simulink library "takeoffToLandingOpenWater_cl"  (R2020a)
settings: Solver=VariableStepAuto  StartTime=0.0  StopTime=10.0  RelTol=1e-3
undefined symbols (not defined in the file or in its folder): a, courseFollow, courseFollow_cl, desiredMoment, elvDeflLaunch, elvDeflStrt, env, exit, FLIGHTCONTROLLER, fltCtrl, freqRollYaw, gain2to3, gain4to1, initializeBussesFromBlock, maxTether, minTether, pathEnable, pathFollowingController, pathFollowingController_cl, peakElevation, phase2Elevator, rollAmp, rollCtrlKd, rollCtrlKp, rollCtrlTau, rollPhase, rollYawPeriod, takeOffToLandingExp, tsSpool, vhcl, xcurrent, yawAmp, yawCtrlKd, yawCtrlKp, yawPhase
libraries: simulink x4, filteredPIDController_ul x4, angleBtw2Vecs_ul x4, dspsigops x3, pathGeometry_ul x3, ctrlAllocMatrix3Comp_cl x2, setpointToOutput_cl x2, tanFrameProjection_ul x2, vectorNormalizer_ul x2, velocityAngle_ul x2, findClosestPointOnPath_new x1, eulAng2RotMat_ul x1
(part 2 of 2)

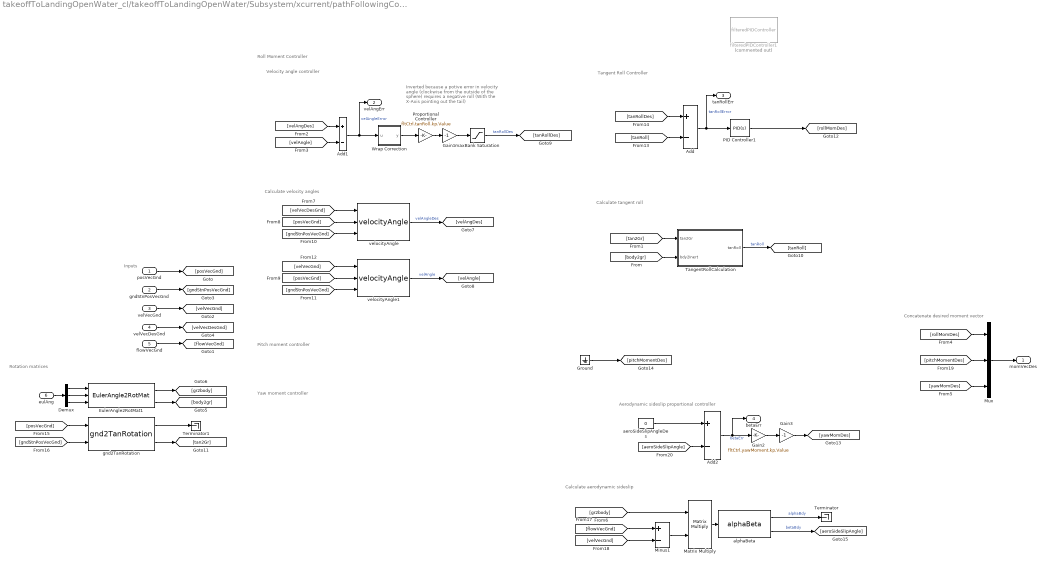
== system takeoffToLandingOpenWater_cl/takeoffToLandingOpenWater/Subsystem/xcurrent/pathFollowingController/desiredMoment ==
  note: Yaw moment controller
  note: Pitch moment controller
  note: Inverted because a potive error
      | in velocity angle (clockwise from the
      | outside of the sphere) requires a negative
      | roll (With the X-Axis pointing out the tail)
  note: Velocity angle controller
  note: Inputs
  note: Rotation matrices
  note: Calculate velocity angles
  note: Calculate tangent roll
  note: Tangent Roll Controller
  note: Concatenate desired moment vector
  note: Roll Moment Controller
  note: Aerodynamic sideslip proportional controller
  note: Calculate aerodynamic sideslip
  posVecGnd : Inport
  gndStnPosVecGnd : Inport  Port=2
  velVecGnd : Inport  Port=3
  velVecDesGnd : Inport  Port=4
  flowVecGnd : Inport  Port=5
  eulAng : Inport  Port=6
  Add : Sum  Inputs=+-
  Add1 : Sum  Inputs=+-
  Add2 : Sum  Inputs=+-
  Demux : Demux  Outputs=3
  EulerAngle2RotMat1 : eulAng2RotMat_ul/EulerAngle2RotMat  SystemSampleTime=-1  Latency=0  AutoFrameSizeCalculation=off
  Gain1 : Gain  Gain=-1
  Gain2 : Gain  Gain=fltCtrl.yawMoment.kp.Value
  Gain3 : Gain  Gain=-1
  Ground : Ground
  Matrix Multiply : Product  Multiplication=Matrix(*)
  Minus1 : Sum  Inputs=+-
  Mux : Mux  Inputs=3
  PID Controller1 : simulink/Continuous/PID Controller  Controller=PID  Form=Parallel  TimeDomain=Continuous-time  UseExternalTs=off  SampleTime=-1  IntegratorMethod=Forward Euler  FilterMethod=Forward Euler  ControllerParametersSource=internal  P=pathCtrl.rollMoment.kp.Value  I=0  D=pathCtrl.rollMoment.kd.Value  UseFilter=on  N=100  TunerSelectOption=Transfer Function Based (PID Tuner App)  InitialConditionSource=internal  InitialConditionForIntegrator=0  InitialConditionForFilter=0  DifferentiatorICPrevScaledInput=0  ExternalReset=none  TrackingMode=off  Kt=1  LimitOutput=off  UpperSaturationLimit=inf  LowerSaturationLimit=-inf  LinearizeAsGain=on  AntiWindupMode=none  Kb=1  POutMin=[]  POutMax=[]  IOutMin=[]  IOutMax=[]  DOutMin=[]  DOutMax=[]  NOutMin=[]  NOutMax=[]  SumOutMin=[]  SumOutMax=[]  SaturationOutMin=[]  SaturationOutMax=[]  PParamMin=[]  PParamMax=[]  IParamMin=[]  IParamMax=[]  DParamMin=[]  DParamMax=[]  NParamMin=[]  NParamMax=[]  KbParamMin=[]  KbParamMax=[]  KtParamMin=[]  KtParamMax=[]  KbOutMin=[]  KbOutMax=[]  KtOutMin=[]  KtOutMax=[]  IntegratorOutMin=[]  IntegratorOutMax=[]  FilterOutMin=[]  FilterOutMax=[]  SumI1OutMin=[]  SumI1OutMax=[]  SumI2OutMin=[]  SumI2OutMax=[]  SumI3OutMin=[]  SumI3OutMax=[]  SumI4OutMin=[]  SumI4OutMax=[]  SumDOutMin=[]  SumDOutMax=[]  DifferentiatorOutMin=[]  DifferentiatorOutMax=[]  FilterDiffOutCoefMin=[]  FilterDiffOutCoefMax=[]  ReciprocalOutMin=[]  ReciprocalOutMax=[]  SumDenOutMin=[]  SumDenOutMax=[]  SumNumOutMin=[]  SumNumOutMax=[]  DivideOutMin=[]  DivideOutMax=[]  UdiffTsProdOutMin=[]  UdiffTsProdOutMax=[]  NTsProdOutMin=[]  NTsProdOutMax=[]  UintegralTsProdOutMin=[]  UintegralTsProdOutMax=[]  UngainTsProdOutMin=[]  UngainTsProdOutMax=[]  IntegratorContinuousStateAttributes=''  IntegratorStateMustResolveToSignalObject=off  IntegratorRTWStateStorageClass=Auto  FilterContinuousStateAttributes=''  FilterStateMustResolveToSignalObject=off  FilterRTWStateStorageClass=Auto  ParallelPVariant=InternalParameters  IdealPVariant=Disabled  IVariant=InternalParameters  DVariant=InternalParameters  IntegratorVariant=Continuous  SatVariant=Disabled  AWVariant=Passthrough  PCopyVariant=Disabled  TRVariant=Disabled  FdbkBlocksVariant=Forward  IdealPFdbkVariant=Disabled  SatFdbkVariant=Disabled  DerivativeFilterVariant=ContFilter  NVariant=InternalParameters  NCopyVariant=Disabled  FilterICVariant=InternalICsFilter  IntegratorICVariant=InternalICs  ExternalResetVariant=Disabled  TRSumVariant=Passthrough  SumFdbkVariant=Disabled  SumVariant=Sum_PID  TsampFilterVariant=InternalTs  TsampNgainVariant=Passthrough  TsampIntegralVariant=Passthrough
  Proportional Controller : Gain  Gain=fltCtrl.tanRoll.kp.Value
  TangentRollCalculation : Subsystem
  Terminator : Terminator
  Terminator1 : Terminator
  Wrap Correction : Subsystem
  aeroSideSlipAngleDes : Constant  Value=0
  alphaBeta : alphaBeta_ul/alphaBeta  SystemSampleTime=-1  Latency=0  AutoFrameSizeCalculation=off
  filteredPIDController1 : filteredPIDController_ul/filteredPIDController  Commented=on  kp=pathCtrl.rollMoment.kp.Value  ki=0  kd=pathCtrl.rollMoment.kd.Value  Value=pathCtrl.rollMoment.tau.Value  externalReset=none
  gnd2TanRotation : gnd2TanRotation_ul/gnd2TanRotation  SystemSampleTime=-1  Latency=0  AutoFrameSizeCalculation=off
  maxBank Saturation : Saturate  UpperLimit=pathCtrl.maxBank.upperLimit.Value  LowerLimit=pathCtrl.maxBank.lowerLimit.Value
  velocityAngle : velocityAngle_ul/velocityAngle  SystemSampleTime=-1  Latency=0  AutoFrameSizeCalculation=off
  velocityAngle1 : velocityAngle_ul/velocityAngle  SystemSampleTime=-1  Latency=0  AutoFrameSizeCalculation=off
  momVecDes : Outport  VectorParamsAs1DForOutWhenUnconnected=off
  velAngErr : Outport  Port=2
  tanRollErr : Outport  Port=3
  betaErr : Outport  Port=4
  wires:
  PID Controller1/1 -> [rollMomDes]
  [pitchMomentDes] -> Mux/2
  Ground/1 -> [pitchMomentDes]
  [aeroSideSlipAngle] -> Add2/2
  [yawMomDes] -> Mux/3
  [rollMomDes] -> Mux/1
  gnd2TanRotation/1 -> Terminator1/1
  gnd2TanRotation/2 -> [tan2Gr]
  [gndStnPosVecGnd] -> gnd2TanRotation/2
  [posVecGnd] -> gnd2TanRotation/1
  [tanRollDes] -> Add/1
  [tanRoll] -> Add/2
  [velVecGnd] -> velocityAngle1/1
  [gndStnPosVecGnd] -> velocityAngle1/3
  [gndStnPosVecGnd] -> velocityAngle/3
  [posVecGnd] -> velocityAngle1/2
  [posVecGnd] -> velocityAngle/2
  [velVecDesGnd] -> velocityAngle/1
  [velAngle] -> Add1/2
  [velAngDes] -> Add1/1
  velocityAngle1/1 -> [velAngle]  "velAngle"
  velocityAngle/1 -> [velAngDes]  "velAngleDes"
  velVecDesGnd/1 -> [velVecDesGnd]
  gndStnPosVecGnd/1 -> [gndStnPosVecGnd]
  alphaBeta/1 -> Terminator/1  "alphaBdy"
  Gain3/1 -> [yawMomDes]
  Mux/1 -> momVecDes/1
  aeroSideSlipAngleDes/1 -> Add2/1
  Add2/1 -> Gain2/1, betaErr/1  "betaErr"
  alphaBeta/2 -> [aeroSideSlipAngle]  "betaBdy"
  Matrix Multiply/1 -> alphaBeta/1
  [gr2body] -> Matrix Multiply/1
  [body2gr] -> TangentRollCalculation/2(bdy2Inert)
  EulerAngle2RotMat1/1 -> [gr2body]
  EulerAngle2RotMat1/2 -> [body2gr]
  Demux/2 -> EulerAngle2RotMat1/2
  Demux/1 -> EulerAngle2RotMat1/1
  Demux/3 -> EulerAngle2RotMat1/3
  eulAng/1 -> Demux/1
  [flowVecGnd] -> Minus1/1
  [velVecGnd] -> Minus1/2
  Minus1/1 -> Matrix Multiply/2
  Gain2/1 -> Gain3/1
  TangentRollCalculation/1(tanRoll) -> [tanRoll]  "tanRoll"
  [tan2Gr] -> TangentRollCalculation/1(tan2Gr)
  flowVecGnd/1 -> [flowVecGnd]
  Add1/1 -> Wrap Correction/1(u), velAngErr/1  "velAngleError"
  maxBank Saturation/1 -> [tanRollDes]  "tanRollDes"
  Gain1/1 -> maxBank Saturation/1
  Proportional Controller/1 -> Gain1/1
  Wrap Correction/1(y) -> Proportional Controller/1
  Add/1 -> PID Controller1/1, tanRollErr/1  "tanRollError"
  velVecGnd/1 -> [velVecGnd]
  posVecGnd/1 -> [posVecGnd]

== system takeoffToLandingOpenWater_cl/takeoffToLandingOpenWater/Subsystem/xcurrent/pathFollowingController/courseFollow/GoldenSectionPathSearch ==
  lastKnownS : Inport
  pathParams : Inport  Port=2
  currentPos : Inport  Port=3
  pathCntr : Inport  Port=4
  From11 : From  Commented=on  GotoTag=geomParams
  From27 : From  Commented=on  GotoTag=pathCntr
  From28 : From  Commented=on  GotoTag=pos
  From30 : From  Commented=on  GotoTag=sPrev
  GoldenSectionMATLAB : MATLAB Function  Commented=on  TreatAsAtomicUnit=on  mask{geomFunc=pathCtrl, searchWidth=0.1, pathVarTol=1e-5}
  GoldenSectionSimulink : Subsystem
  Goto1 : Goto  Commented=on  GotoTag=sStar
  sStar : Outport  InitialOutput=pathCtrl.initPathVar.Value  VectorParamsAs1DForOutWhenUnconnected=off
  wires:
  GoldenSectionSimulink/1(Out1) -> [sStar]
  [sPrev] -> GoldenSectionSimulink/4(sPrev)
  [pathCntr] -> GoldenSectionSimulink/3(cntrPtPosVec)
  [geomParams] -> GoldenSectionSimulink/2(geomParams)
  [pos] -> GoldenSectionSimulink/1(posVecGnd)
  [sStar] -> sStar/1
  lastKnownS/1 -> [sPrev]
  From27/1 -> GoldenSectionMATLAB/3(pathCntrPosVecGnd)
  From30/1 -> GoldenSectionMATLAB/2(sPrev)
  From28/1 -> GoldenSectionMATLAB/1(posVec)
  From11/1 -> GoldenSectionMATLAB/4(geomParams)
  GoldenSectionMATLAB/1(sNext) -> Goto1/1
  pathCntr/1 -> [pathCntr]
  pathParams/1 -> [geomParams]
  currentPos/1 -> [pos]

== system takeoffToLandingOpenWater_cl/takeoffToLandingOpenWater/Subsystem/xcurrent/pathFollowingController/courseFollow/Overwrite Radius ==
  note: subsystem overwrites the 5th basis parameter with the current radius
      | so that the downstream blocks calculate the path geomatry at the current radius.
  pathParamsIn : Inport
  positionVec : Inport  Port=2
  gndStnPos : Inport  Port=3
  Add : Sum  Inputs=+-
  Assignment : Assignment  NumberOfDimensions=2  DiagnosticForDimensions=Warning  IndexOptions=Index vector (dialog),Assign all  Indices=5,5  OutputSizes=1,1
  Dot Product : DotProduct  InputSameDT=on  OutDataTypeStr=Inherit: Inherit via internal rule
  Sqrt : Sqrt  SaturateOnIntegerOverflow=on
  pathParamsOut : Outport  VectorParamsAs1DForOutWhenUnconnected=off
  wires:
  gndStnPos/1 -> Add/2
  positionVec/1 -> Add/1
  pathParamsIn/1 -> Assignment/1
  Sqrt/1 -> Assignment/2
  Assignment/1 -> pathParamsOut/1
  Dot Product/1 -> Sqrt/1
  Add/1 -> Dot Product/1, Dot Product/2

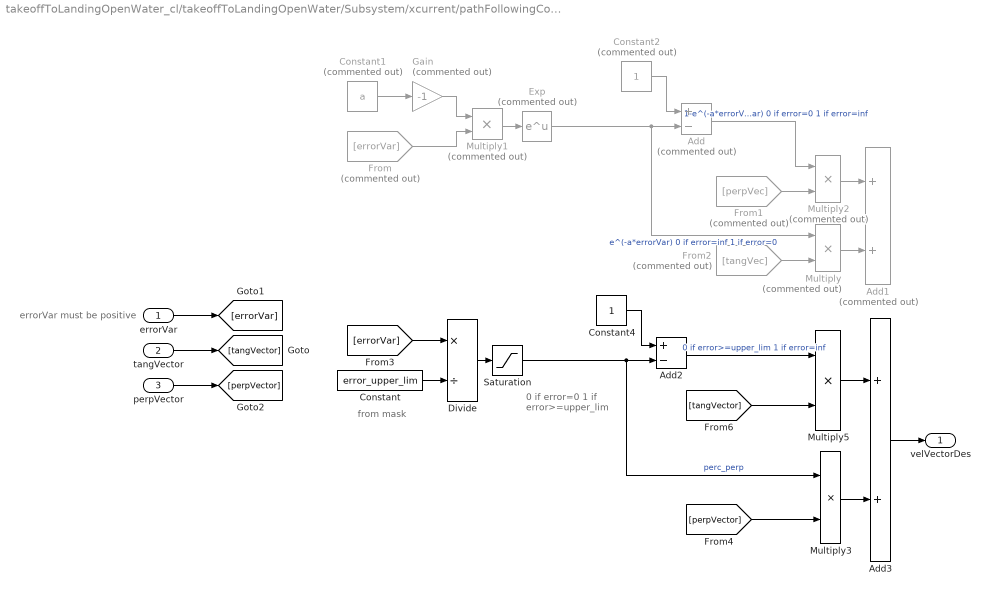
== system takeoffToLandingOpenWater_cl/takeoffToLandingOpenWater/Subsystem/xcurrent/pathFollowingController/courseFollow/saturatedWeightedAverage ==
  note: 0 if error=0
      | 1 if error>=upper_lim
  note: from mask
  note: errorVar must be positive
  "errorVar " : Inport
  tangVector : Inport  Port=2
  "perpVector " : Inport  Port=3
  Add : Sum  Commented=on  Inputs=+-
  Add1 : Sum  Commented=on
  Add2 : Sum  Inputs=+-
  Add3 : Sum
  Constant : Constant  Value=error_upper_lim
  Constant1 : Constant  Commented=on  Value=a
  Constant2 : Constant  Commented=on
  Constant4 : Constant
  Divide : Product  Inputs=*/
  Exp : Math  Commented=on  SignedPower=on  SaturateOnIntegerOverflow=on
  From : From  Commented=on  GotoTag=errorVar
  From1 : From  Commented=on  GotoTag=perpVec
  From2 : From  Commented=on  GotoTag=tangVec
  Gain : Gain  Commented=on  Gain=-1
  Multiply : Product  Commented=on
  Multiply1 : Product  Commented=on
  Multiply2 : Product  Commented=on
  Multiply3 : Product
  Multiply5 : Product
  Saturation : Saturate  UpperLimit=1  LowerLimit=0
  "velVectorDes " : Outport  VectorParamsAs1DForOutWhenUnconnected=off
  wires:
  tangVector/1 -> [tangVector]
  Constant1/1 -> Gain/1
  Gain/1 -> Multiply1/1
  Multiply1/1 -> Exp/1
  Exp/1 -> Multiply/1, Add/2  "e^(-a*errorVar) 0 if error=inf 1 if error=0"
  Constant2/1 -> Add/1
  Add/1 -> Multiply2/1  "1-e^(-a*errorVar) 0 if error=0 1 if error=inf"
  "errorVar "/1 -> [errorVar]
  "perpVector "/1 -> [perpVector]
  From/1 -> Multiply1/2
  Multiply2/1 -> Add1/1
  Multiply/1 -> Add1/2
  From1/1 -> Multiply2/2
  From2/1 -> Multiply/2
  Constant4/1 -> Add2/1
  Saturation/1 -> Multiply3/1, Add2/2  "perc_perp"
  Add3/1 -> "velVectorDes "/1
  Multiply3/1 -> Add3/2
  Multiply5/1 -> Add3/1
  Add2/1 -> Multiply5/1  "0 if error>=upper_lim 1 if error=inf"
  [errorVar] -> Divide/1
  Constant/1 -> Divide/2
  Divide/1 -> Saturation/1
  [tangVector] -> Multiply5/2
  [perpVector] -> Multiply3/2

== system takeoffToLandingOpenWater_cl/takeoffToLandingOpenWater/Subsystem/xcurrent/pathFollowingController/desiredMoment/TangentRollCalculation ==
  note: Angle between body X and tangent Z
  note: Inverted because the right wing
      | being <90deg from Local down
      | is a negative roll about the +X axis
  note: Angle between body Y and tangent Z
  note: Measuring tangent roll as the opposite
      | of the angle between the Body Y axis
      | and the tangent plane
  tan2Gr : Inport
  bdy2Inert : Inport  Port=2
  Constant1 : Constant  Value=pi/2
  Constant2 : Constant  Value=pi/2
  Constant3 : Constant  Value=[0 1 0]'
  Constant4 : Constant  Value=[0 0 1]'
  Constant5 : Constant  Value=[1 0 0]'
  Constant6 : Constant  Value=[0 0 1]'
  Gain : Gain  Gain=-1
  Matrix Multiply{,1..3} (4 alike) : Product  Multiplication=Matrix(*)
  Subtract : Sum  Inputs=+-
  Subtract1 : Sum  Inputs=+-
  Terminator : Terminator
  angleBtw2DVecs : angleBtw2Vecs_ul/angleBtw2DVecs  SystemSampleTime=-1  Latency=0  AutoFrameSizeCalculation=off
  angleBtw2DVecs1 : Subsystem
  tanRoll : Outport  VectorParamsAs1DForOutWhenUnconnected=off
  wires:
  Constant5/1 -> Matrix Multiply2/2
  angleBtw2DVecs1/1(angle) -> Subtract1/2
  Constant1/1 -> Subtract1/1
  Matrix Multiply3/1 -> angleBtw2DVecs1/1(vec1)
  Constant6/1 -> Matrix Multiply3/2
  Matrix Multiply2/1 -> angleBtw2DVecs1/2(vec2)
  tan2Gr/1 -> Matrix Multiply1/1, Matrix Multiply3/1
  Subtract1/1 -> Terminator/1  "tanPitch"
  bdy2Inert/1 -> Matrix Multiply/1, Matrix Multiply2/1
  Gain/1 -> tanRoll/1  "tanRoll"
  Subtract/1 -> Gain/1
  Matrix Multiply/1 -> angleBtw2DVecs/2
  Constant4/1 -> Matrix Multiply1/2
  Matrix Multiply1/1 -> angleBtw2DVecs/1
  Constant2/1 -> Subtract/1
  angleBtw2DVecs/1 -> Subtract/2
  Constant3/1 -> Matrix Multiply/2

== system takeoffToLandingOpenWater_cl/takeoffToLandingOpenWater/Subsystem/xcurrent/pathFollowingController/desiredMoment/Wrap Correction ==
  note: output = mod(input-pi,2*pi)-pi
      | wraps output to -pi to pi
      |
      | ex) 1.5*pi will become -.5pi
      | 	and -1.5pi will become .5pi
      |
      | to visualize, plot the fuction above
  u : Inport
  Add1 : Sum  Inputs=+-
  Add2 : Sum  Inputs=+-
  Constant1 : Constant  Value=pi
  Constant2 : Constant  Value=2*pi
  Constant3 : Constant  Value=pi
  Mod : Math  Operator=mod  SignedPower=on  SaturateOnIntegerOverflow=on
  y : Outport  VectorParamsAs1DForOutWhenUnconnected=off
  wires:
  Add2/1 -> y/1
  Constant3/1 -> Add2/2
  Mod/1 -> Add2/1  "always_pos"
  Constant2/1 -> Mod/2
  Add1/1 -> Mod/1
  Constant1/1 -> Add1/2
  u/1 -> Add1/1

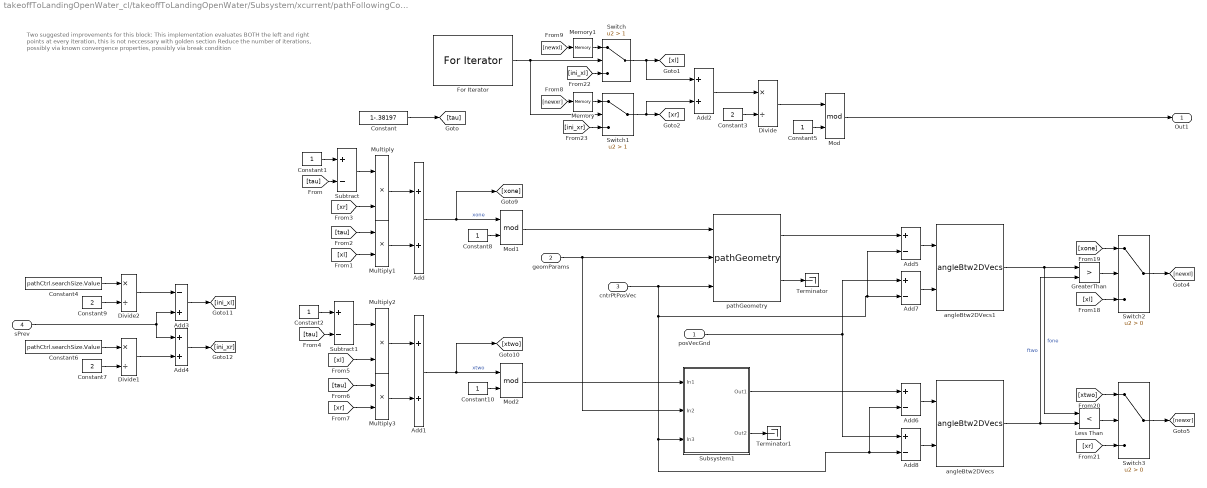
== system takeoffToLandingOpenWater_cl/takeoffToLandingOpenWater/Subsystem/xcurrent/pathFollowingController/courseFollow/GoldenSectionPathSearch/GoldenSectionSimulink ==
  note: Two suggested improvements for this block:
      | This implementation evaluates BOTH the left and right points at every iteration, this is not neccessary with golden section
      | Reduce the number of iterations, possibly via known convergence properties, possibly via break condition
  posVecGnd : Inport
  geomParams : Inport  Port=2
  cntrPtPosVec : Inport  Port=3
  sPrev : Inport  Port=4
  Add{,1..2,4} (4 alike) : Sum
  Add3 : Sum  Inputs=-+
  Add{5..8} (4 alike) : Sum  Inputs=+-
  Constant : Constant  Value=1-.38197
  Constant{1..2,5,8,10} (5 alike) : Constant
  Constant3 : Constant  Value=2
  Constant4 : Constant  Value=pathCtrl.searchSize.Value
  Constant6 : Constant  Value=pathCtrl.searchSize.Value
  Constant7 : Constant  Value=2
  Constant9 : Constant  Value=2
  Divide : Product  Inputs=*/
  Divide1 : Product  Inputs=*/
  Divide2 : Product  Inputs=*/
  For Iterator : ForIterator  IterationLimit=25
  GreaterThan : RelationalOperator  Operator=>  OutDataTypeStr=boolean  RndMeth=Simplest
  Less Than : RelationalOperator  Operator=<  OutDataTypeStr=boolean  RndMeth=Simplest
  Memory : Memory  InheritSampleTime=on
  Memory1 : Memory  InheritSampleTime=on
  Mod : Math  Operator=mod  SignedPower=on  SaturateOnIntegerOverflow=on
  Mod1 : Math  Operator=mod  SignedPower=on  SaturateOnIntegerOverflow=on
  Mod2 : Math  Operator=mod  SignedPower=on  SaturateOnIntegerOverflow=on
  Multiply{,1..3} (4 alike) : Product
  Subsystem1 : Subsystem
  Subtract : Sum  Inputs=+-
  Subtract1 : Sum  Inputs=+-
  Switch : Switch  Criteria=u2 > Threshold  Threshold=1
  Switch1 : Switch  Criteria=u2 > Threshold  Threshold=1
  Switch2 : Switch  Criteria=u2 > Threshold
  Switch3 : Switch  Criteria=u2 > Threshold
  Terminator : Terminator
  Terminator1 : Terminator
  angleBtw2DVecs : angleBtw2Vecs_ul/angleBtw2DVecs  SystemSampleTime=-1  Latency=0  AutoFrameSizeCalculation=off
  angleBtw2DVecs1 : angleBtw2Vecs_ul/angleBtw2DVecs  SystemSampleTime=-1  Latency=0  AutoFrameSizeCalculation=off
  pathGeometry : pathGeometry_ul/pathGeometry  SystemSampleTime=-1  Latency=0  AutoFrameSizeCalculation=off
  Out1 : Outport
  wires:
  Add8/1 -> angleBtw2DVecs/2
  Multiply1/1 -> Add/2
  Switch3/1 -> [newxr]
  [ini_xl] -> Switch/3
  Mod/1 -> Out1/1
  Divide2/1 -> Add3/1
  Switch2/1 -> [newxl]
  pathGeometry/2 -> Terminator/1
  [newxl] -> Memory1/1
  Constant6/1 -> Divide1/1
  Add6/1 -> angleBtw2DVecs/1
  Constant10/1 -> Mod2/2
  Add2/1 -> Divide/1
  [xl] -> Switch2/3
  [xr] -> Switch3/3
  Divide/1 -> Mod/1
  [xl] -> Multiply2/2
  Multiply3/1 -> Add1/2
  Add5/1 -> angleBtw2DVecs1/1
  sPrev/1 -> Add3/2, Add4/1
  Less Than/1 -> Switch3/2
  Constant3/1 -> Divide/2
  Add4/1 -> [ini_xr]
  Constant9/1 -> Divide2/2
  [xr] -> Multiply/2
  Add3/1 -> [ini_xl]
  Divide1/1 -> Add4/2
  Mod1/1 -> pathGeometry/1
  Memory/1 -> Switch1/1
  [newxr] -> Memory/1
  Add7/1 -> angleBtw2DVecs1/2
  [tau] -> Multiply1/1
  [xone] -> Switch2/1
  [ini_xr] -> Switch1/3
  angleBtw2DVecs1/1 -> GreaterThan/1, Less Than/1  "fone"
  Constant4/1 -> Divide2/1
  Mod2/1 -> Subsystem1/1(In1)
  Multiply2/1 -> Add1/1
  Switch1/1 -> [xr], Add2/2
  Constant/1 -> [tau]
  Add/1 -> Mod1/1, [xone]  "xone"
  For Iterator/1 -> Switch/2, Switch1/2
  Memory1/1 -> Switch/1
  [tau] -> Multiply3/1
  [tau] -> Subtract/2
  [xtwo] -> Switch3/1
  Multiply/1 -> Add/1
  [xl] -> Multiply1/2
  Subsystem1/2(Out2) -> Terminator1/1
  Subtract/1 -> Multiply/1
  Constant7/1 -> Divide1/2
  Add1/1 -> Mod2/1, [xtwo]  "xtwo"
  [tau] -> Subtract1/2
  angleBtw2DVecs/1 -> Less Than/2, GreaterThan/2  "ftwo"
  Constant5/1 -> Mod/2
  Constant1/1 -> Subtract/1
  posVecGnd/1 -> Add7/1, Add8/1
  GreaterThan/1 -> Switch2/2
  pathGeometry/1 -> Add5/1
  Constant8/1 -> Mod1/2
  [xr] -> Multiply3/2
  Subsystem1/1(Out1) -> Add6/1
  Constant2/1 -> Subtract1/1
  geomParams/1 -> Subsystem1/2(In2), pathGeometry/2
  Switch/1 -> [xl], Add2/1
  cntrPtPosVec/1 -> pathGeometry/3, Add7/2, Add5/2, Subsystem1/3(In3), Add8/2, Add6/2
  Subtract1/1 -> Multiply2/1

== system takeoffToLandingOpenWater_cl/takeoffToLandingOpenWater/Subsystem/xcurrent/pathFollowingController/desiredMoment/TangentRollCalculation/angleBtw2DVecs1 ==
  vec1 : Inport
  vec2 : Inport  Port=2
  Abs : Abs
  Atan2 : Trigonometry  Operator=atan2
  Cross Product : vrlib/Utilities/Cross Product
      settings: SourceProductBaseCode=VR
  Dot Product : DotProduct  InputSameDT=on  OutDataTypeStr=Inherit: Inherit via internal rule
  Dot Product1 : DotProduct  InputSameDT=on  OutDataTypeStr=Inherit: Inherit via internal rule
  Sqrt : Sqrt  SaturateOnIntegerOverflow=on
  angle : Outport  VectorParamsAs1DForOutWhenUnconnected=off
  wires:
  Sqrt/1 -> Atan2/1
  Dot Product1/1 -> Sqrt/1
  Abs/1 -> angle/1
  Dot Product/1 -> Atan2/2
  Cross Product/1 -> Dot Product1/2, Dot Product1/1
  vec2/1 -> Dot Product/2, Cross Product/1
  vec1/1 -> Cross Product/2, Dot Product/1
  Atan2/1 -> Abs/1

== system takeoffToLandingOpenWater_cl/takeoffToLandingOpenWater/Subsystem/xcurrent/pathFollowingController/courseFollow/GoldenSectionPathSearch/GoldenSectionSimulink/Subsystem1 ==
  In1 : Inport
  In2 : Inport  Port=2
  In3 : Inport  Port=3
  pathGeometry : pathGeometry_ul/pathGeometry  SystemSampleTime=-1  Latency=0  AutoFrameSizeCalculation=off
  Out1 : Outport  VectorParamsAs1DForOutWhenUnconnected=off
  Out2 : Outport  Port=2  VectorParamsAs1DForOutWhenUnconnected=off
  wires:
  pathGeometry/2 -> Out2/1
  In1/1 -> pathGeometry/1
  In3/1 -> pathGeometry/3
  pathGeometry/1 -> Out1/1
  In2/1 -> pathGeometry/2

== matlab function takeoffToLandingOpenWater_cl/takeoffToLandingOpenWater/Subsystem/xcurrent/pathFollowingController/MATLAB Function3 ==
  data: r input; basisParams output
function basisParams = fcn(r)

h = 2*asin(2/2/r );  w = 2*asin(6/2/r );                              %   rad - Path width/height
[a,b] = boothParamConversion(w,h);

basisParams = [a,b,-deg2rad(35),180*pi/180,r-.1];

== matlab function takeoffToLandingOpenWater_cl/takeoffToLandingOpenWater/Subsystem/xcurrent/pathFollowingController/courseFollow/GoldenSectionPathSearch/GoldenSectionMATLAB ==
  data: posVec input; sNext output; sPrev input; pathCntrPosVecGnd input; pathVarTol parameter; searchWidth parameter; geomParams input
function sNext = fcn(posVec,sPrev,pathCntrPosVecGnd, pathVarTol, searchWidth, geomParams)
% I wrote this function on 4/22/2020 when attempting to figure out some
% issues with numerical stiffness.  Turns out that althought the profiler
% was telling me the problem was with the simulink in the equivalent
% subsystem, that was a lie.  Anyways, I thought I should leave this here
% anyways just in case anyone wants to reference it.  Note that this
% implementation doesn't allow for different paths without changing
% function J below.  Which isn't great for a long term solution, so don't
% just use this as-is if you want to go to a matlab-based golden section
% implementation in the future. Also, I think there are some hard-coded
% numbers in the mask in the model, so fix that.  Finally, note that even
% though the "equivalent" simulink implementation has some inefficiencies
% that this code doesnt (as noted in the simulink implementation), there
% doesn't appear to be a siginificant difference in run times, although I
% haven't done a thorough study. -Mitchell

% phi = (sqrt(5) + 1) / 2;
% gr = 1/((1/phi)+1);
% gr = 0.618033988749895;
x1 = sPrev - searchWidth/2;
x4 = sPrev + searchWidth/2;
x2 = x4 - (x4-x1)*0.618033988749895;
x3 = x1 + (x4-x1)*0.618033988749895;
% J1 = J(x1,posVec,geomParams,pathCntrPosVecGnd);
J2 = J(x2,posVec,geomParams,pathCntrPosVecGnd);
J3 = J(x3,posVec,geomParams,pathCntrPosVecGnd);
% J4 = J(x4,posVec,geomParams,pathCntrPosVecGnd);
% JL =JFunc(xL);
% JR = JFunc(xR);
% plot([x1 x2 x3 x4],[J1 J2 J3 J4])
for ii = 1:100 
    if J2<J3
        x4 = x3;
%         J4 = J(x4,posVec,geomParams,pathCntrPosVecGnd);
        x3 = x2;
        J3 = J2;
        x2 = x4 - (x4-x1)*0.618033988749895;
        J2 = J(x2,posVec,geomParams,pathCntrPosVecGnd);
    else
        x1 = x2;
%         J1 = J(x1,posVec,geomParams,pathCntrPosVecGnd);
        x2 = x3;
        J2 = J3;
        x3 = x1 + (x4-x1)*0.618033988749895;
        J3 = J(x3,posVec,geomParams,pathCntrPosVecGnd);
    end
    if x4-x1<pathVarTol/2
        break
    end
end
sNext = mod((x4+x1)/2,1);
end

function val = J(sTest,posVec,geomParams,pathCntr)
az = atan2(posVec(2),posVec(1));
el = atan2(posVec(3),sqrt(posVec(1)^2+posVec(2)^2));
pathPosVec = lemOfBooth(sTest,geomParams,pathCntr);
azP = atan2(pathPosVec(2),pathPosVec(1));
elP = atan2(pathPosVec(3),sqrt(pathPosVec(1)^2+pathPosVec(2)^2));
val = (az-azP)^2+(el-elP)^2;
end

== matlab function takeoffToLandingOpenWater_cl/takeoffToLandingOpenWater/Subsystem/MATLAB Function ==
  data: state input; trig output
function trig = fcn(state)
trig = 0; 
if state ==3
trig = 1; 
end

== matlab function takeoffToLandingOpenWater_cl/takeoffToLandingOpenWater/Subsystem/xcurrent/pathFollowingController/MATLAB Function ==
  data: t input; y output; freqRollYaw input; rollPhase input; rollAmp input
function y = fcn(t,freqRollYaw,rollPhase,rollAmp)

y = rollAmp*sin(freqRollYaw*t + rollPhase) +180;

== matlab function takeoffToLandingOpenWater_cl/takeoffToLandingOpenWater/Subsystem/xcurrent/pathFollowingController/MATLAB Function1 ==
  data: t input; y output; freqRollYaw input; yawPhase input; yawAmp input
function y = fcn(t,freqRollYaw,yawPhase,yawAmp)

y = yawAmp*sin(freqRollYaw*t + yawPhase);

== stateflow chart takeoffToLandingOpenWater_cl/takeoffToLandingOpenWater/Chart ==
  state init
    boolVec=[0 1 0 0];
  state non_x
    boolVec=[1 0 0 0];
  state exit
    boolVec=[0 0 0 1];
  state cross
    boolVec=[0 0 1 0];
  (default) -> non_x
  non_x -> init : [and(and(and(r <minTL,velMag < flowVelMag ),time >150),elevation < elvPeak)]
  exit -> non_x : [velMag < .8*flowVelMag*gain41]
  init -> cross : [velMag > flowVelMag*gain23]
  cross -> exit : [r > maxR]
  data: boolVec output; r input; velMag input; flowVelMag input; maxR parameter; pathVar input; elevation input; elevationLast input; time input; gain41 parameter; gain23 parameter; minTL parameter; elvPeak parameter

== matlab function takeoffToLandingOpenWater_cl/takeoffToLandingOpenWater/Subsystem/xcurrent/pathFollowingController/MATLAB Function2 ==
  data: t input; v_sp output
function v_sp   = fcn(t)
v_sp = 0;




if t< 15 || t>150
    v_sp = 0;
else
    v_sp = .001*(t-15)^2;
end
